simulink model "radar_af"  (R2019a)
settings: Solver=ode45  StartTime=0.0  StopTime=T-Ts  RelTol=1e-3  EnableMultiTasking=on
undefined symbols (not defined in the file or in its folder): f0, t1, td, Tram, Ts, var
libraries: simulink x1
settings Model: Creator=Jachu  LastModifiedBy=ASUS_PEPE
settings DataIOCC: SaveFormat=StructureWithTime  SignalLoggingSaveFormat=ModelDataLogs  ReturnWorkspaceOutputs=off
settings OptimizationCC: LifeSpan=inf
settings DebuggingCC: FcnCallInpInsideContextMsg=warning  SFUnexpectedBacktrackingDiag=warning  SFNoUnconditionalDefaultTransitionDiag=warning  SFExecutionAtInitializationDiag=none  ArithmeticOperatorsInVariantConditions=warning
settings HardwareCC: ProdBitPerPointer=32  ProdBitPerSizeT=32  ProdBitPerPtrDiffT=32  ProdLargestAtomicFloat=None  ProdWordSize=32  ProdHWDeviceType=Specified
settings ModelReferenceCC: PropagateSignalLabelsOutOfModel=off
settings SFSimCC: SimUseLocalCustomCode=off
settings RTWCC: RTWUseLocalCustomCode=off
settings CodeAppCC: StateflowObjectComments=on
settings GRTTargetCC: TargetLangStandard=C89/C90 (ANSI)  GeneratePreprocessorConditionals=Disable all  CombineOutputUpdateFcns=off  GRTInterface=on
settings ConfigComp: CovMetricSettings=dw  CovHtmlReporting=on  CovSaveCumulativeToWorkspaceVar=on  CovSaveSingleToWorkspaceVar=on  CovExternalEMLEnable=off

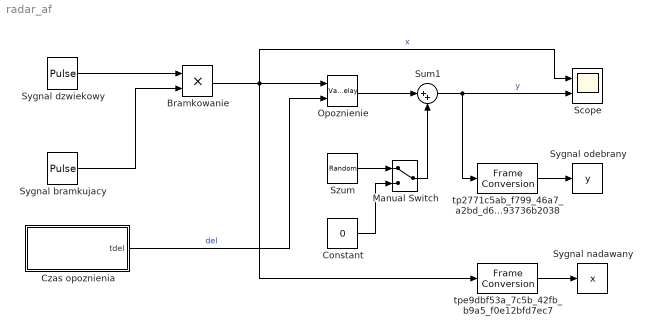
== system radar_af ==
  Bramkowanie : Product
  Constant : Constant  Value=0
  Czas opoznienia : Subsystem
  Manual Switch : ManualSwitch
  Opoznienie : VariableTransportDelay  VariableDelayType=Variable transport delay  MaximumDelay=10  MaximumPoints=2000000
  Scope : Scope  NumInputPorts=2
  Sum1 : Sum  Inputs=|++
  Sygnal bramkujacy : DiscretePulseGenerator  PulseType=Time based  Period=Tram  PulseWidth=t1
  Sygnal dzwiekowy : DiscretePulseGenerator  PulseType=Time based  Period=1/f0  PulseWidth=25
  Sygnal nadawany : ToWorkspace  VariableName=x  SampleTime=Ts
  Sygnal odebrany : ToWorkspace  VariableName=y  SampleTime=Ts
  Szum : RandomNumber  Variance=var  Seed=13  SampleTime=Ts
  tp2771c5ab_f799_46a7_a2bd_d693736b2038 : FrameConversion  OutFrame=Sample-based
  tpe9dbf53a_7c5b_42fb_b9a5_f0e12bfd7ec7 : FrameConversion  OutFrame=Sample-based
  wires:
  Sygnal dzwiekowy/1 -> Bramkowanie/1
  Bramkowanie/1 -> tpe9dbf53a_7c5b_42fb_b9a5_f0e12bfd7ec7/1, Scope/1, Opoznienie/1  "x"
  Opoznienie/1 -> Sum1/1
  Sum1/1 -> Scope/2, tp2771c5ab_f799_46a7_a2bd_d693736b2038/1  "y"
  Sygnal bramkujacy/1 -> Bramkowanie/2
  Czas opoznienia/1(tdel) -> Opoznienie/2  "del"
  tpe9dbf53a_7c5b_42fb_b9a5_f0e12bfd7ec7/1 -> Sygnal nadawany/1
  tp2771c5ab_f799_46a7_a2bd_d693736b2038/1 -> Sygnal odebrany/1
  Szum/1 -> Manual Switch/1
  Manual Switch/1 -> Sum1/2
  Constant/1 -> Manual Switch/2

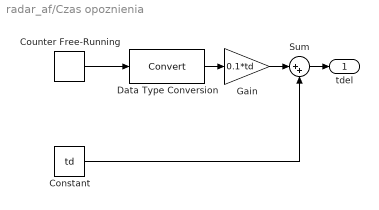
== system radar_af/Czas opoznienia ==
  Constant : Constant  Value=td
  Counter Free-Running : simulink/Sources/Counter Free-Running  NumBits=8  tsamp=Tram
  Data Type Conversion : DataTypeConversion  RndMeth=Round
  Gain : Gain  Gain=0.1*td  OutDataTypeStr=double
  Sum : Sum  Inputs=|++
  tdel : Outport
  wires:
  Data Type Conversion/1 -> Gain/1
  Constant/1 -> Sum/2
  Gain/1 -> Sum/1
  Counter Free-Running/1 -> Data Type Conversion/1
  Sum/1 -> tdel/1
